simulink model "servos"  (R2020a)
settings: Solver=VariableStepAuto  StartTime=0.0  StopTime=10  RelTol=1e-3
values from neighbouring files (symbols this model uses):
  K1 = K(:,1:4)    [servo.m]
  K2 = K(:,5:6)    [servo.m]
  L = real(L)    [servo.m]
  y_sp = [0.4;0.8]    [servo.m]
undefined symbols (not defined in the file or in its folder): A, B, C
settings Model: Creator=wyton  LastModifiedBy=wyton

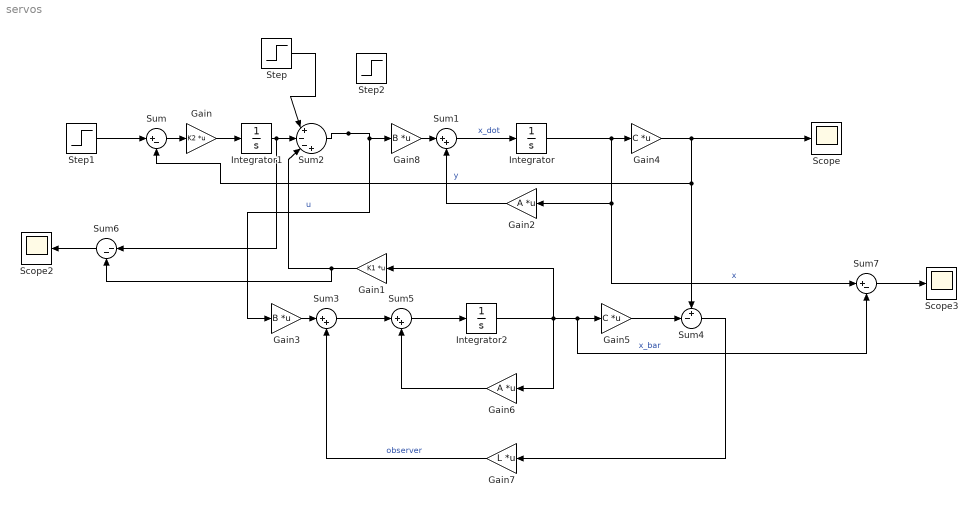
== system servos ==
  Gain : Gain  Gain=K2  Multiplication=Matrix(K*u)
  Gain1 : Gain  Gain=K1  Multiplication=Matrix(K*u)
  Gain2 : Gain  Gain=A  Multiplication=Matrix(K*u)
  Gain3 : Gain  Gain=B  Multiplication=Matrix(K*u)
  Gain4 : Gain  Gain=C  Multiplication=Matrix(K*u)
  Gain5 : Gain  Gain=C  Multiplication=Matrix(K*u)
  Gain6 : Gain  Gain=A  Multiplication=Matrix(K*u)
  Gain7 : Gain  Gain=L  Multiplication=Matrix(K*u)
  Gain8 : Gain  Gain=B  Multiplication=Matrix(K*u)
  Integrator : Integrator
  Integrator1 : Integrator
  Integrator2 : Integrator
  Scope : Scope
      settings: AttributesFormatString=output
  Scope2 : Scope
      settings: AttributesFormatString=control signal
  Scope3 : Scope
      settings: AttributesFormatString=estimate error
  Step : Step  Time=10  Before=[0;0]  After=[0;0]  SampleTime=0
      settings: AttributesFormatString=disturbance
  Step1 : Step  Time=0  Before=[0;0]  After=y_sp  SampleTime=0
      settings: AttributesFormatString=set point
  Step2 : Step  Time=0  Before=[0,0]  After=[1,0]  SampleTime=0
  Sum : Sum  Inputs=|+-
  Sum1 : Sum  Inputs=|++
  Sum2 : Sum  Inputs=|+--+
  Sum3 : Sum  Inputs=|++
  Sum4 : Sum  Inputs=+-|
  Sum5 : Sum  Inputs=|++
  Sum6 : Sum  Inputs=|--
  Sum7 : Sum  Inputs=|+-
  wires:
  Sum1/1 -> Integrator/1  "x_dot"
  Gain2/1 -> Sum1/2
  Integrator/1 -> Gain2/1, Sum7/1, Gain4/1  "x"
  Gain4/1 -> Sum4/1, Sum/2, Scope/1  "y"
  Gain3/1 -> Sum3/1
  Sum3/1 -> Sum5/1
  Sum5/1 -> Integrator2/1
  Integrator2/1 -> Gain5/1, Sum7/2, Gain1/1, Gain6/1  "x_bar"
  Gain6/1 -> Sum5/2
  Gain5/1 -> Sum4/2
  Gain7/1 -> Sum3/2  "observer"
  Sum4/1 -> Gain7/1
  Gain1/1 -> Sum2/3, Sum6/2
  Gain8/1 -> Sum1/1
  Sum2/1 -> Gain8/1, Gain3/1  "u"
  Sum/1 -> Gain/1
  Gain/1 -> Integrator1/1
  Integrator1/1 -> Sum2/2, Sum6/1
  Step/1 -> Sum2/1
  Sum6/1 -> Scope2/1
  Sum7/1 -> Scope3/1
  Step1/1 -> Sum/1
